simulink model "FLIGHT_Hexacopter_V2_1"  (R2024a)
settings: Solver=FixedStepDiscrete  StartTime=0.0  StopTime=inf  FixedStep=SampleTime_SAS  RelTol=1e-3  EnableMultiTasking=on
InitFcn:
  | Init_FLIGHT_Hexacopter
values from neighbouring files (symbols this model uses):
  d2r = pi/180    (= 0.0174532925199)    [Init_FLIGHT_Hexacopter.m]
  Jxx = 0.0211    [Init_FLIGHT_Hexacopter.m]
  Jyy = 0.0219    [Init_FLIGHT_Hexacopter.m]
  Jzz = 0.0366    [Init_FLIGHT_Hexacopter.m]
  Kpp = 3.3894    [Init_FLIGHT_Hexacopter_fromNCMS.m]
  Kpr = 3.3894    [Init_FLIGHT_Hexacopter_fromNCMS.m]
  MAX_CONTROL_ANGLE_PITCH = 30*pi/180    (= 0.523598775598)    [Init_FLIGHT_Hexacopter.m]    (also in Init_FLIGHT_Hexacopter_fromNCMS.m = 0.349065850399)
  MAX_CONTROL_ANGLE_RATE_PITCH = 360*pi/180    (= 6.28318530718)    [Init_FLIGHT_Hexacopter.m]    (also in Init_FLIGHT_Hexacopter_fromNCMS.m)
  MAX_CONTROL_ANGLE_RATE_ROLL = 360*pi/180    (= 6.28318530718)    [Init_FLIGHT_Hexacopter.m]    (also in Init_FLIGHT_Hexacopter_fromNCMS.m)
  MAX_CONTROL_ANGLE_RATE_Y = 120*pi/180    (= 2.09439510239)    [Init_FLIGHT_Hexacopter.m]    (also in Init_FLIGHT_Hexacopter_fromNCMS.m)
  MAX_CONTROL_ANGLE_ROLL = 30*pi/180    (= 0.523598775598)    [Init_FLIGHT_Hexacopter.m]    (also in Init_FLIGHT_Hexacopter_fromNCMS.m = 0.349065850399)
  MAX_CONTROL_VELOCITY_XY = 1.5    [Init_FLIGHT_Hexacopter.m]    (also in Init_FLIGHT_Hexacopter_fromNCMS.m)
  MAX_CONTROL_VELOCITY_Z = 1    [Init_FLIGHT_Hexacopter.m]    (also in Init_FLIGHT_Hexacopter_fromNCMS.m)
  SampleTime = 1/250    (= 0.004)    [Init_FLIGHT_Hexacopter.m]    (also in Init_FLIGHT_Hexacopter_fromNCMS.m = 0.01)
  SampleTime_SAS = 1/1000    (= 0.001)    [Init_FLIGHT_Hexacopter.m]
undefined symbols (not defined in the file or in its folder): arguments, DiscIntNeverNeededParam, event_sequence, id, log_levels, MPC_Z_D, MPC_Z_I, MPC_Z_P, timestamp
libraries: px4lib x42, simulink x9, px4Utilslib x8, px4uORBlib x8, slpidlib x5, simulink_extras x2, sharedtransform x1, px4Sensorslib x1, matrix_library x1
(part 3 of 3)

== matlab function FLIGHT_Hexacopter_V2_1/OFP/MATLAB Function1 ==
  data: in_roll input double; in_pitch input double; in_yawrate input double; flag input boolean; out_roll output double; out_pitch output double; out_yawrate output double; time_usec input double; peak_angle_deg input double; doublet_dt input double; doublet_axis input int32
function [out_roll, out_pitch,out_yawrate]= DoubletGenerator(in_roll, in_pitch, in_yawrate, flag, time_usec, peak_angle_deg, doublet_dt, doublet_axis)
persistent start_time_usec;
if(isempty(start_time_usec))
    start_time_usec = -1;
end

if(flag && start_time_usec == -1)
    start_time_usec = time_usec;
end
d2r = pi/180;

if (flag && start_time_usec > 0) % time calculation
    reletive_time_sec = double(time_usec - start_time_usec)*1e-6;
else
    start_time_usec = -1;
    reletive_time_sec = 0;
end

% Define Doublet
t1 = 0;
t2 = t1+doublet_dt;
t3 = t2+doublet_dt;
peak_angle_rad = peak_angle_deg * d2r;

% Default Output
out_roll = in_roll;
out_pitch = in_pitch;
out_yawrate = in_yawrate;

% Generate Doublet Command
if(flag)
    if(reletive_time_sec >= t1 && reletive_time_sec < t2)
        cmd = peak_angle_rad;
    elseif(reletive_time_sec >= t2 && reletive_time_sec < t3)
        cmd = -peak_angle_rad;
    else
        cmd = 0;
    end

    switch(double(doublet_axis))
        case 1
            out_roll = cmd;
        case 2
            out_pitch = cmd;
        case 3
            out_yawrate = cmd;
    end
end

== matlab function FLIGHT_Hexacopter_V2_1/OFP/MATLAB Function ==
  data: stab_u input; y output; alt_u input; pos_u input; mode input; flag_pos_mode input; flag_alt_mode input
function y = flightmode(stab_u, alt_u, pos_u, mode, flag_pos_mode, flag_alt_mode)

if(mode >= 1800 && flag_pos_mode) % position
    y = pos_u;
elseif(mode <1800 && mode >=1400 && flag_alt_mode) % Altitude
    y = alt_u;
else % Stablized
    y = stab_u;
end

== matlab function FLIGHT_Hexacopter_V2_1/Read_uORB(250hz)_SENSORS250/quat2eul ==
  data: q input; ypr output
function ypr  = quat2eul(q)

% Quaternion conversion to Euler angles based on the PX4 Firmware v1.10.2
% release.

phi = atan2(2*(q(1)*q(2) + q(3)* q(4)), q(1)^2 - q(2)^2 - q(3)^2 + q(4)^2);
theta = asin(-2*(q(2)*q(4) - q(1)*q(3)));
psi = atan2(2*(q(2)*q(3) + q(1)* q(4)), q(1)^2 + q(2)^2 - q(3)^2 - q(4)^2);

ypr = [psi theta phi];

end

== matlab function FLIGHT_Hexacopter_V2_1/Read_uORB(250hz)_SENSORS250/MATLAB Function ==
  data: nav_stat input; flag_stab output; flag_alt output; flag_pos output
function [flag_stab, flag_alt, flag_pos] = flightmode(nav_stat)

if(nav_stat == 1) % ALT Mode
    flag_pos = false;
    flag_alt = true;
    flag_stab = false;

elseif(nav_stat == 2) % POS Mode
    flag_pos = true;
    flag_alt = false;
    flag_stab = false;

else % STAB mode
    flag_pos = false;
    flag_alt = false;
    flag_stab = true;
end

== matlab function FLIGHT_Hexacopter_V2_1/SCAS/MATLAB Function ==
  data: omega_dot input; omega input; H output; w input; fx input; phi_cmd_ddot input; phi_cmd_dot input; e input; kp input; ki input; kd input
function H = H(omega_dot, omega, w, fx, phi_cmd_ddot, phi_cmd_dot, e, kp,ki,kd)

%phi_cmd_ddot = 0; % Suppose
H = kd*(omega_dot*w + omega*fx - phi_cmd_ddot) + kp*(omega_dot*w - phi_cmd_dot) + ki*e;

== matlab function FLIGHT_Hexacopter_V2_1/SCAS/MATLAB Function1 ==
  data: omega input; G1 output; gx input; kd input
function G1 = G(omega, gx, kd)

G1 = omega * gx*kd;

== matlab function FLIGHT_Hexacopter_V2_1/SCAS/MATLAB Function2 ==
  data: Hx input; u output; G1x input; R input
function u = U(Hx, G1x, R)

G1_inv = pinv(G1x);

u = G1_inv * (-Hx + R);
